simulink model "task1"  (R2022b)
settings: Solver=ode45  StartTime=0.0  StopTime=stoptime  MaxStep=0.01  RelTol=1e-7
values from neighbouring files (symbols this model uses):
  A0 = [1 0 0; 0 1 0; 0 0 1]    [lab6task1m.m]    (also in lab6task2m.m; task1main.m; task2main.m; taskmain.m = vrrotvec2mat(axisangle))
  euler312_0 = [-atan2(A0(2,1),A0(2,2)); asin(A0(2,3)); -atan2(A0(1,3),A0(3,3))]    [lab6task1m.m]    (also in lab6task2m.m; task1main.m; task2main.m; taskmain.m)
  euler313_0 = [-atan2(A0(3,1),A0(3,2)); asin(A0(3,3)); atan2(A0(1,3),A0(2,3))]    [lab6task1m.m]    (also in lab6task2m.m; task1main.m; task2main.m; taskmain.m)
  gamma0 = [0;0;1]    [lab6task1m.m]    (also in lab6task2m.m; task1main.m; task2main.m; taskmain.m = [1;0;0])
  I = diag(I)    [lab6task1m.m]    (also in lab6task2m.m; task1main.m; task2main.m; taskmain.m)
  I_inv = pinv(I)    [lab6task1m.m]    (also in lab6task2m.m; task1main.m; task2main.m; taskmain.m)
  Ir = 0.005    [lab6task1m.m]    (also in lab6task2m.m; task1main.m; task2main.m; taskmain.m)
  k = [0;0;1]    [lab6task1m.m]    (also in lab6task2m.m; task1main.m; task2main.m; taskmain.m)
  M = [0;0;0]    [lab6task1m.m]    (also in lab6task2m.m; task1main.m; task2main.m; taskmain.m)
  Mr = 0    [lab6task1m.m]    (also in lab6task2m.m; task1main.m; task2main.m; taskmain.m)
  n = sqrt(mu_E/(height+R_E)^3)    [lab6task1m.m]    (also in lab6task2m.m; task1main.m; task2main.m)
  q0 = zeros(4,1)    [lab6task1m.m]    (also in lab6task2m.m; task1main.m; task2main.m; taskmain.m)
  w0 = cat(1,w0,wr0)    [lab6task1m.m]    (also in lab6task2m.m; task1main.m; task2main.m; taskmain.m)
  w_LN = [0;0;n]    [lab6task1m.m]    (also in lab6task2m.m; task1main.m; task2main.m)
libraries: matrix_library x3, vrlib x2
settings Model: Creator=a1pab  LastModifiedBy=a1pab

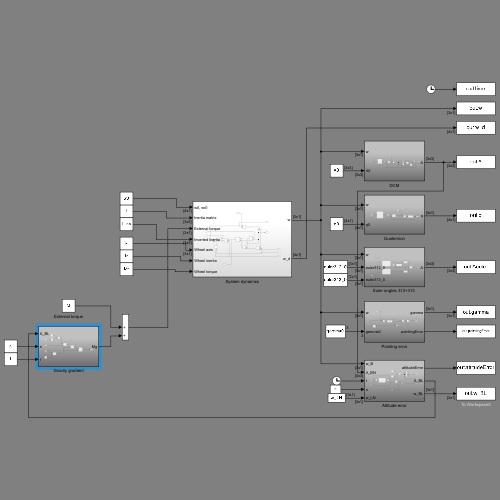
[thumbnail: Simulink's stored preview of the top-level diagram]
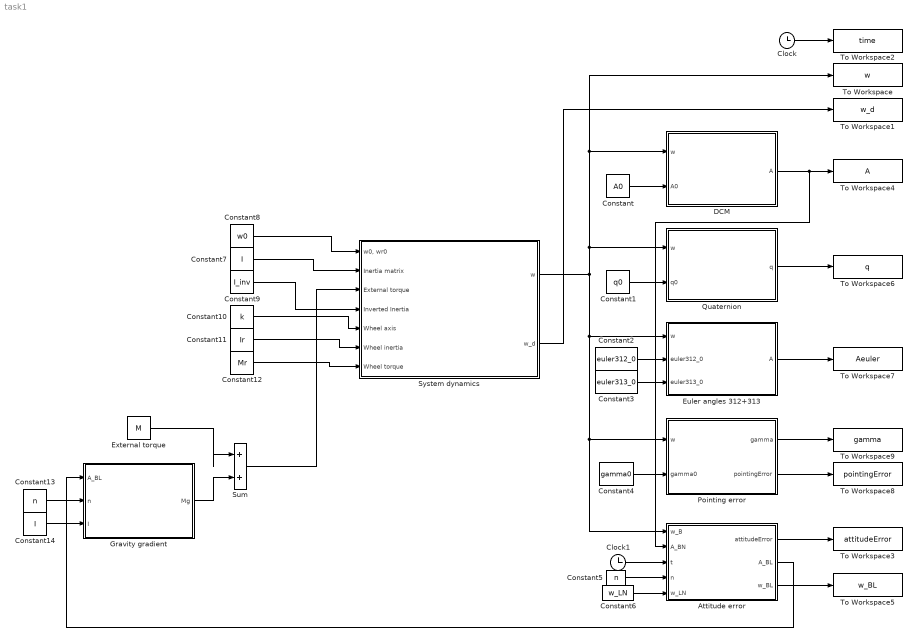
== system task1 ==
  Attitude error : Subsystem
  Clock : Clock
  Clock1 : Clock
  Constant : Constant  Value=A0  VectorParams1D=off
  Constant1 : Constant  Value=q0  VectorParams1D=off
  Constant10 : Constant  Value=k  VectorParams1D=off
  Constant11 : Constant  Value=Ir
  Constant12 : Constant  Value=Mr
  Constant13 : Constant  Value=n  VectorParams1D=off
  Constant14 : Constant  Value=I  VectorParams1D=off
  Constant2 : Constant  Value=euler312_0  VectorParams1D=off
  Constant3 : Constant  Value=euler313_0  VectorParams1D=off
  Constant4 : Constant  Value=gamma0
  Constant5 : Constant  Value=n  VectorParams1D=off
  Constant6 : Constant  Value=w_LN  VectorParams1D=off
  Constant7 : Constant  Value=I  VectorParams1D=off
  Constant8 : Constant  Value=w0  VectorParams1D=off
  Constant9 : Constant  Value=I_inv  VectorParams1D=off
  DCM : Subsystem
  "Euler angles 312+313 " : Subsystem
  External torque : Constant  Value=M
  Gravity gradient : Subsystem
  Pointing error : Subsystem
  Quaternion : Subsystem
  Sum : Sum  Inputs=|++
  System dynamics : Subsystem
  To Workspace : ToWorkspace  VariableName=w  SampleTime=-1
  To Workspace1 : ToWorkspace  VariableName=w_d  SampleTime=-1
  To Workspace2 : ToWorkspace  VariableName=time  SampleTime=-1
  To Workspace3 : ToWorkspace  VariableName=attitudeError  SampleTime=-1
  To Workspace4 : ToWorkspace  VariableName=A  SampleTime=-1
  To Workspace5 : ToWorkspace  VariableName=w_BL  SampleTime=-1
  To Workspace6 : ToWorkspace  VariableName=q  SampleTime=-1
  To Workspace7 : ToWorkspace  VariableName=Aeuler  SampleTime=-1
  To Workspace8 : ToWorkspace  VariableName=pointingError  SampleTime=-1
  To Workspace9 : ToWorkspace  VariableName=gamma  SampleTime=-1
  wires:
  System dynamics/1(w) -> Attitude error/1(w_B), Pointing error/1(w), "Euler angles 312+313 "/1(w), Quaternion/1(w), To Workspace/1, DCM/1(w)
  System dynamics/2(w_d) -> To Workspace1/1
  Clock/1 -> To Workspace2/1
  Constant10/1 -> System dynamics/5(Wheel axis)
  Constant11/1 -> System dynamics/6(Wheel inertia)
  Constant12/1 -> System dynamics/7(Wheel torque)
  Constant8/1 -> System dynamics/1("w0, wr0")
  Constant7/1 -> System dynamics/2(Inertia matrix)
  Constant9/1 -> System dynamics/4(Inverted Inertia)
  Constant/1 -> DCM/2(A0)
  Constant1/1 -> Quaternion/2(q0)
  Quaternion/1(q) -> To Workspace6/1
  Constant2/1 -> "Euler angles 312+313 "/2(euler312_0)
  Constant3/1 -> "Euler angles 312+313 "/3(euler313_0)
  "Euler angles 312+313 "/1(A) -> To Workspace7/1
  Constant4/1 -> Pointing error/2(gamma0)
  Pointing error/2(pointingError) -> To Workspace8/1
  Pointing error/1(gamma) -> To Workspace9/1
  DCM/1(A) -> Attitude error/2(A_BN), To Workspace4/1
  Attitude error/1(attitudeError) -> To Workspace3/1
  Attitude error/3(w_BL) -> To Workspace5/1
  Clock1/1 -> Attitude error/3(t)
  Constant5/1 -> Attitude error/4(n)
  Constant6/1 -> Attitude error/5(w_LN)
  External torque/1 -> Sum/1
  Gravity gradient/1(Mg) -> Sum/2
  Sum/1 -> System dynamics/3(External torque)
  Attitude error/2(A_BL) -> Gravity gradient/1(A_BL)
  Constant13/1 -> Gravity gradient/2(n)
  Constant14/1 -> Gravity gradient/3(I)

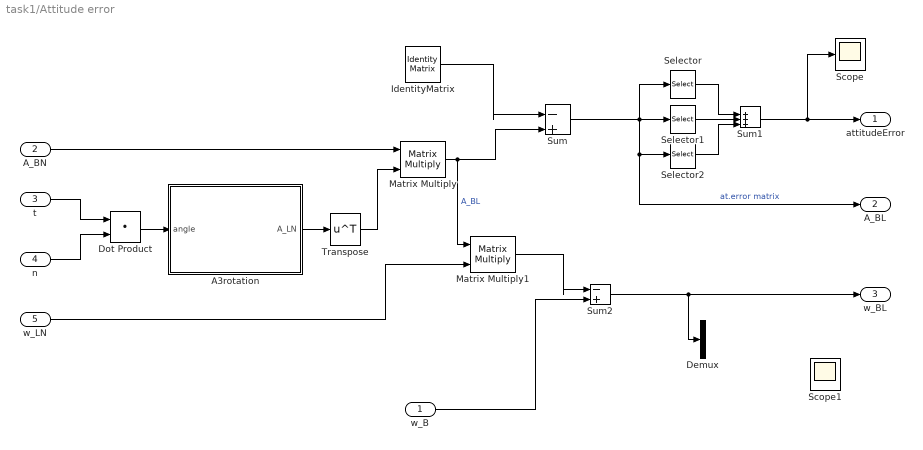
== system task1/Attitude error ==
  w_B : Inport
  A_BN : Inport  Port=2
  t : Inport  Port=3
  n : Inport  Port=4
  w_LN : Inport  Port=5
  A3rotation : Subsystem
  Demux : Demux  Outputs=3
  Dot Product : DotProduct  OutDataTypeStr=Inherit: Inherit via internal rule
  IdentityMatrix : IdentityMatrix  OutputDimensions=3
  Matrix Multiply : Product  Multiplication=Matrix(*)
  Matrix Multiply1 : Product  Multiplication=Matrix(*)
  Scope : Scope
  Scope1 : Scope
  Selector : Selector  NumberOfDimensions=2  InputPortWidth=3  IndexOptions=Index vector (dialog),Index vector (dialog)  Indices=1,1  OutputSizes=1,1
  Selector1 : Selector  NumberOfDimensions=2  InputPortWidth=3  IndexOptions=Index vector (dialog),Index vector (dialog)  Indices=2,2  OutputSizes=1,1
  Selector2 : Selector  NumberOfDimensions=2  InputPortWidth=3  IndexOptions=Index vector (dialog),Index vector (dialog)  Indices=3,3  OutputSizes=1,1
  Sum : Sum  Inputs=|-+
  Sum1 : Sum  Inputs=|+++
  Sum2 : Sum  Inputs=|-+
  Transpose : Math  Operator=transpose
  attitudeError : Outport
  A_BL : Outport  Port=2
  w_BL : Outport  Port=3
  wires:
  t/1 -> Dot Product/1
  n/1 -> Dot Product/2
  Dot Product/1 -> A3rotation/1(angle)
  A3rotation/1(A_LN) -> Transpose/1
  Transpose/1 -> Matrix Multiply/2
  A_BN/1 -> Matrix Multiply/1
  Matrix Multiply/1 -> Matrix Multiply1/1, Sum/2  "A_BL"
  IdentityMatrix/1 -> Sum/1
  Sum/1 -> Selector/1, Selector1/1, A_BL/1, Selector2/1  "at.error matrix"
  Selector/1 -> Sum1/1
  Selector1/1 -> Sum1/2
  Selector2/1 -> Sum1/3
  w_B/1 -> Sum2/2
  Matrix Multiply1/1 -> Sum2/1
  w_LN/1 -> Matrix Multiply1/2
  Sum1/1 -> Scope/1, attitudeError/1
  Sum2/1 -> Demux/1, w_BL/1

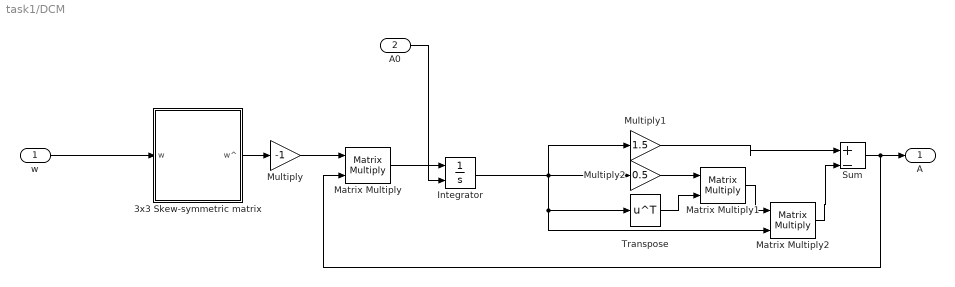
== system task1/DCM ==
  w : Inport
  A0 : Inport  Port=2
  3x3 Skew-symmetric matrix : Subsystem
  Integrator : Integrator  InitialConditionSource=external
  Matrix Multiply : Product  Multiplication=Matrix(*)
  Matrix Multiply1 : Product  Multiplication=Matrix(*)
  Matrix Multiply2 : Product  Multiplication=Matrix(*)
  Multiply : Gain  Gain=-1
  Multiply1 : Gain  Gain=1.5
  Multiply2 : Gain  Gain=0.5
  Sum : Sum  Inputs=|+-
  Transpose : Math  Operator=transpose
  A : Outport
  wires:
  w/1 -> 3x3 Skew-symmetric matrix/1(w)
  3x3 Skew-symmetric matrix/1(w^) -> Multiply/1
  Multiply/1 -> Matrix Multiply/1
  Matrix Multiply/1 -> Integrator/1
  A0/1 -> Integrator/2
  Integrator/1 -> Transpose/1, Matrix Multiply2/2, Multiply2/1, Multiply1/1
  Transpose/1 -> Matrix Multiply1/2
  Sum/1 -> Matrix Multiply/2, A/1
  Matrix Multiply1/1 -> Matrix Multiply2/1
  Matrix Multiply2/1 -> Sum/2
  Multiply1/1 -> Sum/1
  Multiply2/1 -> Matrix Multiply1/1

== system task1/Euler angles 312+313  ==
  w : Inport
  euler312_0 : Inport  Port=2
  euler313_0 : Inport  Port=3
  Abs : Abs  SaturateOnIntegerOverflow=off
  If : If  IfExpression=u1 > 0.1
  If Action Subsystem : Subsystem  TreatAsAtomicUnit=on
  If Action Subsystem1 : Subsystem  TreatAsAtomicUnit=on
  Integrate euler312 : Subsystem
  Integrate euler313 : Subsystem
  Switch : Switch  Criteria=u2 > Threshold  Threshold=0.1  SaturateOnIntegerOverflow=off  InputSameDT=off
  A : Outport
  wires:
  w/1 -> Integrate euler313/1(w), Integrate euler312/1(w)
  euler312_0/1 -> Integrate euler312/2(angles0)
  euler313_0/1 -> Integrate euler313/2(angles0)
  Integrate euler312/2(cos(theta)312) -> Abs/1
  Abs/1 -> Switch/2, If/1
  Integrate euler312/1(euler312) -> If Action Subsystem/1(euler312)
  If/1 -> If Action Subsystem/Action
  Integrate euler313/1(euler313) -> If Action Subsystem1/1(euler313)
  If/2 -> If Action Subsystem1/Action
  If Action Subsystem/1(A) -> Switch/1
  If Action Subsystem1/1(A) -> Switch/3
  Switch/1 -> A/1

== system task1/Gravity gradient ==
  A_BL : Inport
  n : Inport  Port=2
  I : Inport  Port=3
  Constant : Constant  Value=3
  Constant1 : Constant  Value=[1;0;0]  VectorParams1D=off
  Cross Product : matrix_library/Cross Product
  Dot Product : DotProduct  OutDataTypeStr=Inherit: Inherit via internal rule
  Matrix Multiply : Product
  Matrix Multiply1 : Product  Multiplication=Matrix(*)
  Matrix Multiply2 : Product  Multiplication=Matrix(*)
  Square : Math  Operator=square
  Mg : Outport
  wires:
  Constant/1 -> Dot Product/1
  n/1 -> Square/1
  Square/1 -> Dot Product/2
  I/1 -> Matrix Multiply/2
  Dot Product/1 -> Matrix Multiply/1
  Matrix Multiply/1 -> Matrix Multiply1/1
  Matrix Multiply1/1 -> Cross Product/1
  Cross Product/1 -> Mg/1  "3n^2*I*c x c"
  A_BL/1 -> Matrix Multiply2/1
  Constant1/1 -> Matrix Multiply2/2
  Matrix Multiply2/1 -> Cross Product/2, Matrix Multiply1/2  "c"

== system task1/Pointing error ==
  w : Inport
  gamma0 : Inport  Port=2
  Acos : Trigonometry  Operator=acos
  Cross Product : matrix_library/Cross Product
  Dot Product : DotProduct  OutDataTypeStr=Inherit: Inherit via internal rule
  Integrator : Integrator  InitialConditionSource=external
  Normalize Vector : vrlib/Utilities/Normalize Vector  maxzero=0
  gamma : Outport
  pointingError : Outport  Port=2
  wires:
  gamma0/1 -> Dot Product/1, Integrator/2
  w/1 -> Cross Product/2
  Cross Product/1 -> Integrator/1
  Integrator/1 -> Normalize Vector/1
  Normalize Vector/1 -> Dot Product/2, gamma/1, Cross Product/1
  Dot Product/1 -> Acos/1
  Acos/1 -> pointingError/1

== system task1/Quaternion ==
  w : Inport
  q0 : Inport  Port=2
  4x4 Skew-symmetric matrix : Subsystem
  Integrator : Integrator  InitialConditionSource=external
  Matrix Multiply : Product  Multiplication=Matrix(*)
  Multiply : Gain  Gain=0.5
  Normalize Vector : vrlib/Utilities/Normalize Vector  maxzero=0
  q : Outport
  wires:
  w/1 -> 4x4 Skew-symmetric matrix/1(w)
  4x4 Skew-symmetric matrix/1(w^) -> Multiply/1
  Multiply/1 -> Matrix Multiply/1
  Matrix Multiply/1 -> Integrator/1
  q0/1 -> Integrator/2
  Integrator/1 -> Normalize Vector/1
  Normalize Vector/1 -> Matrix Multiply/2, q/1

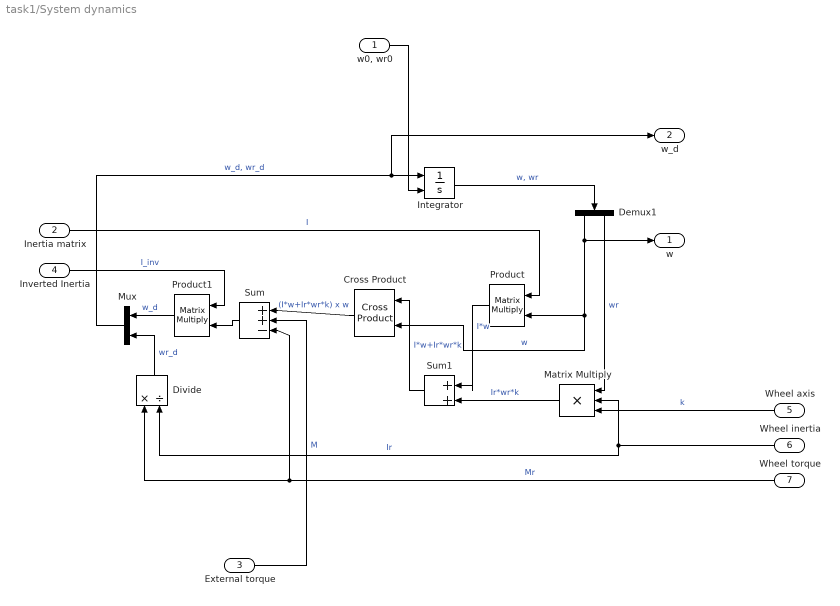
== system task1/System dynamics ==
  "w0, wr0" : Inport
  Inertia matrix : Inport  Port=2
  External torque : Inport  Port=3
  Inverted Inertia : Inport  Port=4
  Wheel axis : Inport  Port=5
  Wheel inertia : Inport  Port=6
  Wheel torque : Inport  Port=7
  Cross Product : matrix_library/Cross Product
  Demux1 : Demux  Outputs=2
  Divide : Product  Inputs=*/
  Integrator : Integrator  InitialConditionSource=external
  Matrix Multiply : Product  Inputs=3
  Mux : Mux  Inputs=2
  Product : Product  Multiplication=Matrix(*)
  Product1 : Product  Multiplication=Matrix(*)
  Sum : Sum  Inputs=|++-
  Sum1 : Sum  Inputs=|++
  w : Outport
  w_d : Outport  Port=2
  wires:
  Mux/1 -> w_d/1, Integrator/1  "w_d, wr_d"
  Integrator/1 -> Demux1/1  "w, wr"
  "w0, wr0"/1 -> Integrator/2
  Product/1 -> Sum1/1  "I*w"
  Cross Product/1 -> Sum/1  "(I*w+Ir*wr*k) x w"
  Inverted Inertia/1 -> Product1/1  "I_inv"
  Inertia matrix/1 -> Product/1  "I"
  Sum/1 -> Product1/2
  External torque/1 -> Sum/2  "M"
  Product1/1 -> Mux/1  "w_d"
  Wheel torque/1 -> Sum/3, Divide/1  "Mr"
  Wheel inertia/1 -> Divide/2, Matrix Multiply/2  "Ir"
  Divide/1 -> Mux/2  "wr_d"
  Demux1/1 -> w/1, Product/2, Cross Product/2  "w"
  Sum1/1 -> Cross Product/1  "I*w+Ir*wr*k"
  Demux1/2 -> Matrix Multiply/1  "wr"
  Matrix Multiply/1 -> Sum1/2  "Ir*wr*k"
  Wheel axis/1 -> Matrix Multiply/3  "k"

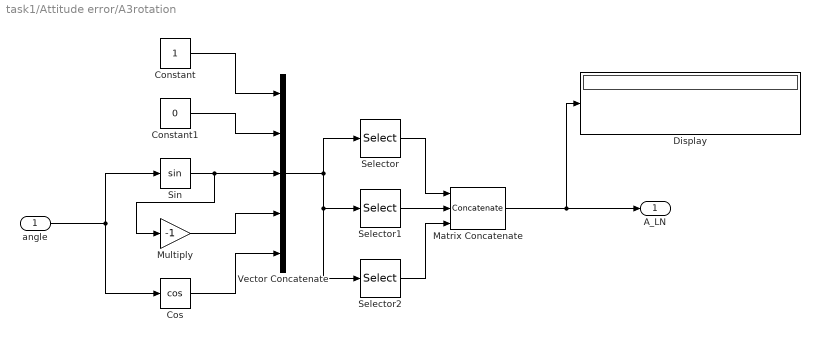
== system task1/Attitude error/A3rotation ==
  angle : Inport
  Constant : Constant
  Constant1 : Constant  Value=0
  Cos : Trigonometry  Operator=cos
  Display : Display
  Matrix Concatenate : Concatenate  NumInputs=3  Mode=Multidimensional array  ConcatenateDimension=2
  Multiply : Gain  Gain=-1
  Selector : Selector  InputPortWidth=5  IndexOptions=Index vector (dialog)  Indices=[5 4 2]  OutputSizes=1
  Selector1 : Selector  InputPortWidth=5  IndexOptions=Index vector (dialog)  Indices=[3 5 2]  OutputSizes=1
  Selector2 : Selector  InputPortWidth=5  IndexOptions=Index vector (dialog)  Indices=[2 2 1]  OutputSizes=1
  Sin : Trigonometry
  Vector Concatenate : Concatenate  NumInputs=5
  A_LN : Outport
  wires:
  angle/1 -> Cos/1, Sin/1
  Sin/1 -> Vector Concatenate/3, Multiply/1
  Constant/1 -> Vector Concatenate/1
  Constant1/1 -> Vector Concatenate/2
  Multiply/1 -> Vector Concatenate/4
  Cos/1 -> Vector Concatenate/5
  Vector Concatenate/1 -> Selector2/1, Selector1/1, Selector/1
  Selector/1 -> Matrix Concatenate/1
  Selector1/1 -> Matrix Concatenate/2
  Selector2/1 -> Matrix Concatenate/3
  Matrix Concatenate/1 -> Display/1, A_LN/1

== system task1/DCM/3x3 Skew-symmetric matrix ==
  w : Inport
  Constant : Constant  Value=0
  Display : Display
  Matrix Concatenate : Concatenate  NumInputs=3  Mode=Multidimensional array  ConcatenateDimension=2
  Multiply : Gain  Gain=-1
  Scope : Scope
  Selector : Selector  InputPortWidth=7  IndexOptions=Index vector (dialog)  Indices=[4 1 5]  OutputSizes=1
  Selector1 : Selector  InputPortWidth=7  IndexOptions=Index vector (dialog)  Indices=[1 7 3]  OutputSizes=1
  Selector2 : Selector  InputPortWidth=7  IndexOptions=Index vector (dialog)  Indices=[6 2 1]  OutputSizes=1
  Transpose : Math  Operator=transpose
  Vector Concatenate : Concatenate  NumInputs=3
  w^ : Outport
  wires:
  Matrix Concatenate/1 -> Transpose/1
  Selector/1 -> Matrix Concatenate/2
  Selector2/1 -> Matrix Concatenate/3
  Selector1/1 -> Matrix Concatenate/1
  Vector Concatenate/1 -> Selector2/1, Selector/1, Selector1/1
  Constant/1 -> Vector Concatenate/1
  w/1 -> Scope/1, Multiply/1, Vector Concatenate/2
  Multiply/1 -> Vector Concatenate/3  "-w"
  Transpose/1 -> Display/1, w^/1

== system task1/Euler angles 312+313 /If Action Subsystem ==
  euler312 : Inport
  Action Port : ActionPort  ActionPortLabel=if(u1 > 0.1)
  A1rotation : Subsystem
  A2rotation : Subsystem
  A3rotation : Subsystem
  Demux : Demux  Outputs=3
  Display : Display
  Matrix Multiply : Product  Inputs=3  Multiplication=Matrix(*)
  A : Outport
  wires:
  euler312/1 -> Demux/1
  Matrix Multiply/1 -> Display/1, A/1
  A2rotation/1(matrix) -> Matrix Multiply/1
  A1rotation/1(matrix) -> Matrix Multiply/2
  A3rotation/1(matrix) -> Matrix Multiply/3
  Demux/1 -> A3rotation/1(angle)
  Demux/2 -> A1rotation/1(angle)
  Demux/3 -> A2rotation/1(angle)

== system task1/Euler angles 312+313 /If Action Subsystem1 ==
  euler313 : Inport
  Action Port : ActionPort  ActionPortLabel=else
  A1rotation : Subsystem
  A3rotation : Subsystem
  A3rotation1 : Subsystem
  Demux : Demux  Outputs=3
  Display : Display
  Matrix Multiply : Product  Inputs=3  Multiplication=Matrix(*)
  A : Outport
  wires:
  euler313/1 -> Demux/1
  A1rotation/1(matrix) -> Matrix Multiply/2
  A3rotation1/1(matrix) -> Matrix Multiply/1
  A3rotation/1(matrix) -> Matrix Multiply/3
  Matrix Multiply/1 -> A/1, Display/1
  Demux/1 -> A3rotation/1(angle)
  Demux/2 -> A1rotation/1(angle)
  Demux/3 -> A3rotation1/1(angle)

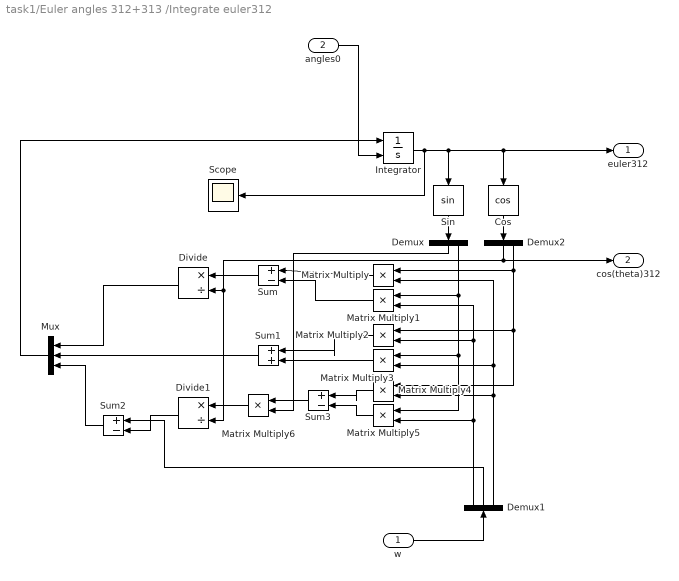
== system task1/Euler angles 312+313 /Integrate euler312 ==
  w : Inport
  angles0 : Inport  Port=2
  Cos : Trigonometry  Operator=cos
  Demux : Demux  Outputs=3
  Demux1 : Demux  Outputs=3
  Demux2 : Demux  Outputs=3
  Divide : Product  Inputs=*/
  Divide1 : Product  Inputs=*/
  Integrator : Integrator  InitialConditionSource=external
  Matrix Multiply{,1..6} (7 alike) : Product
  Mux : Mux  Inputs=3
  Scope : Scope
  Sin : Trigonometry
  Sum : Sum  Inputs=|+-
  Sum1 : Sum  Inputs=|++
  Sum2 : Sum  Inputs=|+-
  Sum3 : Sum  Inputs=|+-
  euler312 : Outport
  cos(theta)312 : Outport  Port=2
  wires:
  w/1 -> Demux1/1
  angles0/1 -> Integrator/2
  Integrator/1 -> Scope/1, Sin/1, Cos/1, euler312/1
  Mux/1 -> Integrator/1
  Sin/1 -> Demux/1
  Cos/1 -> Demux2/1
  Demux1/3 -> Matrix Multiply4/2, Matrix Multiply3/2, Matrix Multiply/2
  Demux2/3 -> Matrix Multiply4/1, Matrix Multiply2/1, Matrix Multiply/1
  Matrix Multiply/1 -> Sum/1
  Demux1/1 -> Matrix Multiply5/2, Matrix Multiply2/2, Matrix Multiply1/2
  Demux/3 -> Matrix Multiply5/1, Matrix Multiply3/1, Matrix Multiply1/1
  Matrix Multiply1/1 -> Sum/2
  Sum/1 -> Divide/1
  Divide/1 -> Mux/1
  Demux2/2 -> cos(theta)312/1, Divide1/2, Divide/2
  Matrix Multiply2/1 -> Sum1/1
  Matrix Multiply3/1 -> Sum1/2
  Sum1/1 -> Mux/2
  Sum2/1 -> Mux/3
  Matrix Multiply4/1 -> Sum3/1
  Matrix Multiply5/1 -> Sum3/2
  Sum3/1 -> Matrix Multiply6/1
  Demux/2 -> Matrix Multiply6/2
  Matrix Multiply6/1 -> Divide1/1
  Divide1/1 -> Sum2/2
  Demux1/2 -> Sum2/1

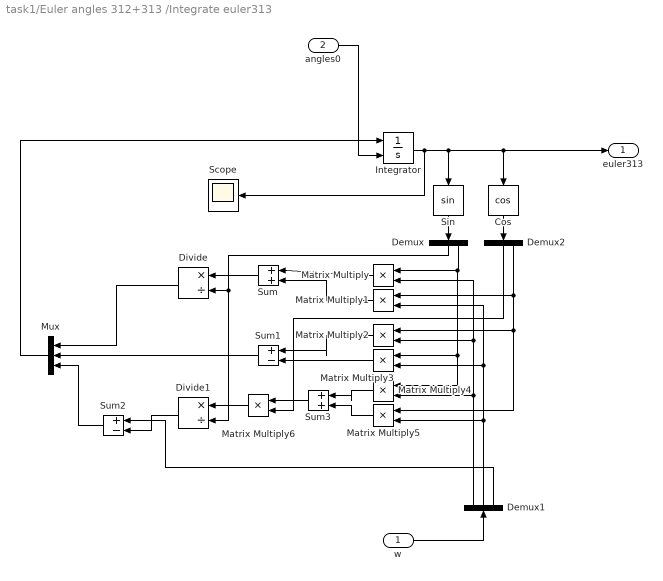
== system task1/Euler angles 312+313 /Integrate euler313 ==
  w : Inport
  angles0 : Inport  Port=2
  Cos : Trigonometry  Operator=cos
  Demux : Demux  Outputs=3
  Demux1 : Demux  Outputs=3
  Demux2 : Demux  Outputs=3
  Divide : Product  Inputs=*/
  Divide1 : Product  Inputs=*/
  Integrator : Integrator  InitialConditionSource=external
  Matrix Multiply{,1..6} (7 alike) : Product
  Mux : Mux  Inputs=3
  Scope : Scope
  Sin : Trigonometry
  Sum : Sum  Inputs=|++
  Sum1 : Sum  Inputs=|+-
  Sum2 : Sum  Inputs=|+-
  Sum3 : Sum  Inputs=|++
  euler313 : Outport
  wires:
  w/1 -> Demux1/1
  Cos/1 -> Demux2/1
  angles0/1 -> Integrator/2
  Sin/1 -> Demux/1
  Integrator/1 -> Scope/1, Sin/1, euler313/1, Cos/1
  Mux/1 -> Integrator/1
  Demux1/1 -> Matrix Multiply4/2, Matrix Multiply2/2, Matrix Multiply/2
  Matrix Multiply/1 -> Sum/1
  Matrix Multiply1/1 -> Sum/2
  Demux1/2 -> Matrix Multiply5/2, Matrix Multiply3/2, Matrix Multiply1/2
  Demux2/3 -> Matrix Multiply5/1, Matrix Multiply2/1, Matrix Multiply1/1
  Sum/1 -> Divide/1
  Demux/2 -> Divide1/2, Divide/2
  Divide/1 -> Mux/1
  Matrix Multiply2/1 -> Sum1/1
  Matrix Multiply3/1 -> Sum1/2
  Sum1/1 -> Mux/2
  Demux/3 -> Matrix Multiply4/1, Matrix Multiply3/1, Matrix Multiply/1
  Matrix Multiply4/1 -> Sum3/1
  Matrix Multiply5/1 -> Sum3/2
  Sum3/1 -> Matrix Multiply6/1
  Demux2/2 -> Matrix Multiply6/2
  Matrix Multiply6/1 -> Divide1/1
  Divide1/1 -> Sum2/2
  Demux1/3 -> Sum2/1
  Sum2/1 -> Mux/3

== system task1/Quaternion/4x4 Skew-symmetric matrix ==
  w : Inport
  Constant : Constant  Value=0
  Display : Display
  Matrix Concatenate : Concatenate  NumInputs=4  Mode=Multidimensional array  ConcatenateDimension=2
  Multiply : Gain  Gain=-1
  Selector : Selector  InputPortWidth=7  IndexOptions=Index vector (dialog)  Indices=[7 1 2 3]  OutputSizes=1
  Selector1 : Selector  InputPortWidth=7  IndexOptions=Index vector (dialog)  Indices=[1 4 6 2]  OutputSizes=1
  Selector2 : Selector  InputPortWidth=7  IndexOptions=Index vector (dialog)  Indices=[3 5 1 4]  OutputSizes=1
  Selector3 : Selector  InputPortWidth=7  IndexOptions=Index vector (dialog)  Indices=[5 6 7 1]  OutputSizes=1
  Transpose : Math  Operator=transpose
  Vector Concatenate : Concatenate  NumInputs=3
  w^ : Outport
  wires:
  Matrix Concatenate/1 -> Transpose/1
  Selector/1 -> Matrix Concatenate/2
  Selector2/1 -> Matrix Concatenate/3
  Selector1/1 -> Matrix Concatenate/1
  Vector Concatenate/1 -> Selector3/1, Selector2/1, Selector/1, Selector1/1
  Constant/1 -> Vector Concatenate/1
  w/1 -> Multiply/1, Vector Concatenate/2
  Multiply/1 -> Vector Concatenate/3  "-w"
  Selector3/1 -> Matrix Concatenate/4
  Transpose/1 -> Display/1, w^/1

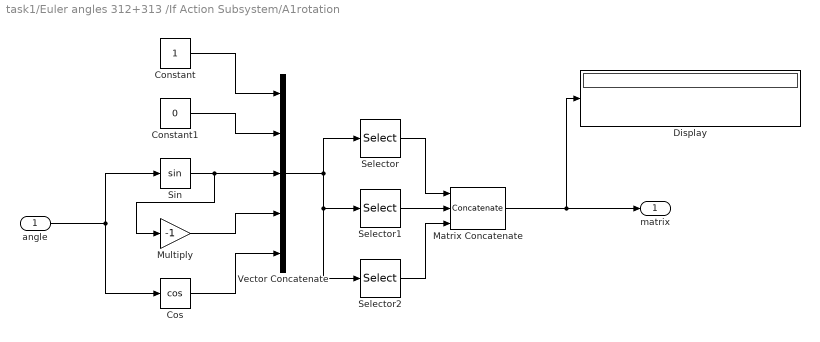
== system task1/Euler angles 312+313 /If Action Subsystem/A1rotation ==
  angle : Inport
  Constant : Constant
  Constant1 : Constant  Value=0
  Cos : Trigonometry  Operator=cos
  Display : Display
  Matrix Concatenate : Concatenate  NumInputs=3  Mode=Multidimensional array  ConcatenateDimension=2
  Multiply : Gain  Gain=-1
  Selector : Selector  InputPortWidth=5  IndexOptions=Index vector (dialog)  Indices=[1 2 2]  OutputSizes=1
  Selector1 : Selector  InputPortWidth=5  IndexOptions=Index vector (dialog)  Indices=[2 5 4]  OutputSizes=1
  Selector2 : Selector  InputPortWidth=5  IndexOptions=Index vector (dialog)  Indices=[2 3 5]  OutputSizes=1
  Sin : Trigonometry
  Vector Concatenate : Concatenate  NumInputs=5
  matrix : Outport
  wires:
  angle/1 -> Cos/1, Sin/1
  Sin/1 -> Vector Concatenate/3, Multiply/1
  Constant/1 -> Vector Concatenate/1
  Constant1/1 -> Vector Concatenate/2
  Multiply/1 -> Vector Concatenate/4
  Cos/1 -> Vector Concatenate/5
  Vector Concatenate/1 -> Selector2/1, Selector1/1, Selector/1
  Selector/1 -> Matrix Concatenate/1
  Selector1/1 -> Matrix Concatenate/2
  Selector2/1 -> Matrix Concatenate/3
  Matrix Concatenate/1 -> Display/1, matrix/1

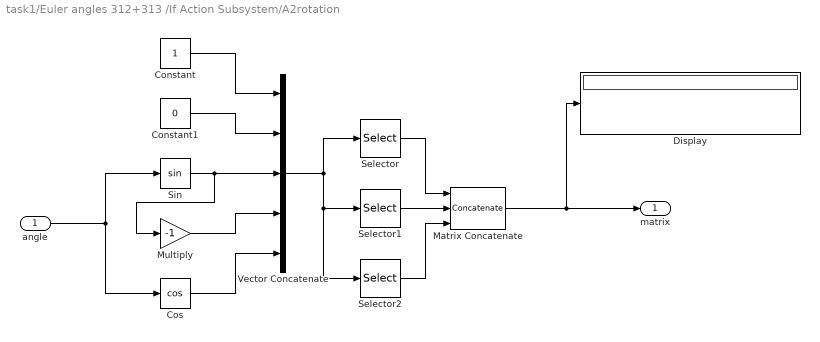
== system task1/Euler angles 312+313 /If Action Subsystem/A2rotation ==
  angle : Inport
  Constant : Constant
  Constant1 : Constant  Value=0
  Cos : Trigonometry  Operator=cos
  Display : Display
  Matrix Concatenate : Concatenate  NumInputs=3  Mode=Multidimensional array  ConcatenateDimension=2
  Multiply : Gain  Gain=-1
  Selector : Selector  InputPortWidth=5  IndexOptions=Index vector (dialog)  Indices=[5 2 3]  OutputSizes=1
  Selector1 : Selector  InputPortWidth=5  IndexOptions=Index vector (dialog)  Indices=[2 1 2]  OutputSizes=1
  Selector2 : Selector  InputPortWidth=5  IndexOptions=Index vector (dialog)  Indices=[4 2 5]  OutputSizes=1
  Sin : Trigonometry
  Vector Concatenate : Concatenate  NumInputs=5
  matrix : Outport
  wires:
  angle/1 -> Cos/1, Sin/1
  Sin/1 -> Vector Concatenate/3, Multiply/1
  Constant/1 -> Vector Concatenate/1
  Constant1/1 -> Vector Concatenate/2
  Multiply/1 -> Vector Concatenate/4
  Cos/1 -> Vector Concatenate/5
  Vector Concatenate/1 -> Selector2/1, Selector1/1, Selector/1
  Selector/1 -> Matrix Concatenate/1
  Selector1/1 -> Matrix Concatenate/2
  Selector2/1 -> Matrix Concatenate/3
  Matrix Concatenate/1 -> Display/1, matrix/1

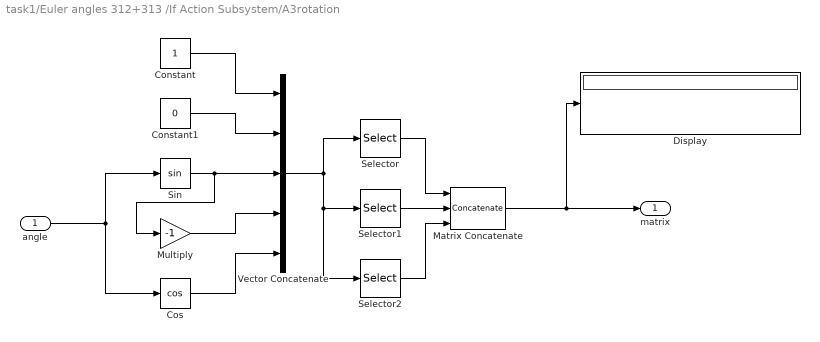
== system task1/Euler angles 312+313 /If Action Subsystem/A3rotation ==
  angle : Inport
  Constant : Constant
  Constant1 : Constant  Value=0
  Cos : Trigonometry  Operator=cos
  Display : Display
  Matrix Concatenate : Concatenate  NumInputs=3  Mode=Multidimensional array  ConcatenateDimension=2
  Multiply : Gain  Gain=-1
  Selector : Selector  InputPortWidth=5  IndexOptions=Index vector (dialog)  Indices=[5 4 2]  OutputSizes=1
  Selector1 : Selector  InputPortWidth=5  IndexOptions=Index vector (dialog)  Indices=[3 5 2]  OutputSizes=1
  Selector2 : Selector  InputPortWidth=5  IndexOptions=Index vector (dialog)  Indices=[2 2 1]  OutputSizes=1
  Sin : Trigonometry
  Vector Concatenate : Concatenate  NumInputs=5
  matrix : Outport
  wires:
  angle/1 -> Cos/1, Sin/1
  Sin/1 -> Vector Concatenate/3, Multiply/1
  Constant/1 -> Vector Concatenate/1
  Constant1/1 -> Vector Concatenate/2
  Multiply/1 -> Vector Concatenate/4
  Cos/1 -> Vector Concatenate/5
  Vector Concatenate/1 -> Selector2/1, Selector1/1, Selector/1
  Selector/1 -> Matrix Concatenate/1
  Selector1/1 -> Matrix Concatenate/2
  Selector2/1 -> Matrix Concatenate/3
  Matrix Concatenate/1 -> Display/1, matrix/1

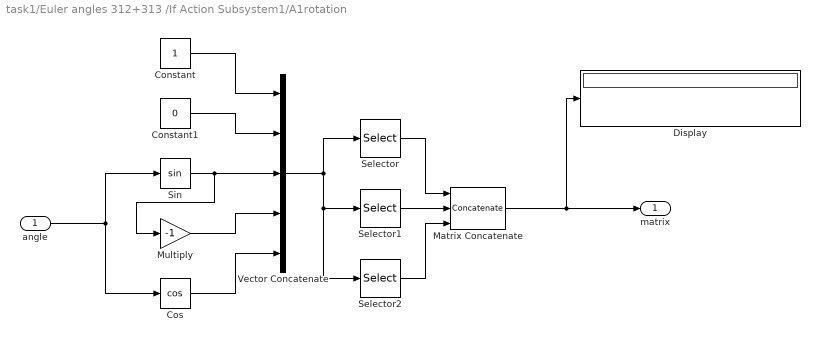
== system task1/Euler angles 312+313 /If Action Subsystem1/A1rotation ==
  angle : Inport
  Constant : Constant
  Constant1 : Constant  Value=0
  Cos : Trigonometry  Operator=cos
  Display : Display
  Matrix Concatenate : Concatenate  NumInputs=3  Mode=Multidimensional array  ConcatenateDimension=2
  Multiply : Gain  Gain=-1
  Selector : Selector  InputPortWidth=5  IndexOptions=Index vector (dialog)  Indices=[1 2 2]  OutputSizes=1
  Selector1 : Selector  InputPortWidth=5  IndexOptions=Index vector (dialog)  Indices=[2 5 4]  OutputSizes=1
  Selector2 : Selector  InputPortWidth=5  IndexOptions=Index vector (dialog)  Indices=[2 3 5]  OutputSizes=1
  Sin : Trigonometry
  Vector Concatenate : Concatenate  NumInputs=5
  matrix : Outport
  wires:
  angle/1 -> Cos/1, Sin/1
  Sin/1 -> Vector Concatenate/3, Multiply/1
  Constant/1 -> Vector Concatenate/1
  Constant1/1 -> Vector Concatenate/2
  Multiply/1 -> Vector Concatenate/4
  Cos/1 -> Vector Concatenate/5
  Vector Concatenate/1 -> Selector2/1, Selector1/1, Selector/1
  Selector/1 -> Matrix Concatenate/1
  Selector1/1 -> Matrix Concatenate/2
  Selector2/1 -> Matrix Concatenate/3
  Matrix Concatenate/1 -> Display/1, matrix/1

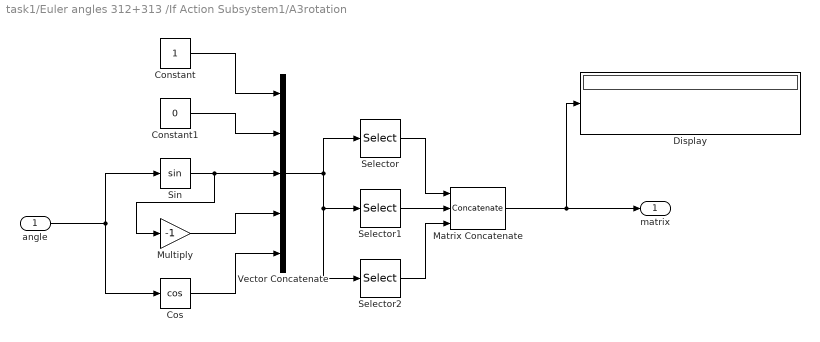
== system task1/Euler angles 312+313 /If Action Subsystem1/A3rotation ==
  angle : Inport
  Constant : Constant
  Constant1 : Constant  Value=0
  Cos : Trigonometry  Operator=cos
  Display : Display
  Matrix Concatenate : Concatenate  NumInputs=3  Mode=Multidimensional array  ConcatenateDimension=2
  Multiply : Gain  Gain=-1
  Selector : Selector  InputPortWidth=5  IndexOptions=Index vector (dialog)  Indices=[5 4 2]  OutputSizes=1
  Selector1 : Selector  InputPortWidth=5  IndexOptions=Index vector (dialog)  Indices=[3 5 2]  OutputSizes=1
  Selector2 : Selector  InputPortWidth=5  IndexOptions=Index vector (dialog)  Indices=[2 2 1]  OutputSizes=1
  Sin : Trigonometry
  Vector Concatenate : Concatenate  NumInputs=5
  matrix : Outport
  wires:
  angle/1 -> Cos/1, Sin/1
  Sin/1 -> Vector Concatenate/3, Multiply/1
  Constant/1 -> Vector Concatenate/1
  Constant1/1 -> Vector Concatenate/2
  Multiply/1 -> Vector Concatenate/4
  Cos/1 -> Vector Concatenate/5
  Vector Concatenate/1 -> Selector2/1, Selector1/1, Selector/1
  Selector/1 -> Matrix Concatenate/1
  Selector1/1 -> Matrix Concatenate/2
  Selector2/1 -> Matrix Concatenate/3
  Matrix Concatenate/1 -> Display/1, matrix/1

== system task1/Euler angles 312+313 /If Action Subsystem1/A3rotation1 ==
  angle : Inport
  Constant : Constant
  Constant1 : Constant  Value=0
  Cos : Trigonometry  Operator=cos
  Display : Display
  Matrix Concatenate : Concatenate  NumInputs=3  Mode=Multidimensional array  ConcatenateDimension=2
  Multiply : Gain  Gain=-1
  Selector : Selector  InputPortWidth=5  IndexOptions=Index vector (dialog)  Indices=[5 4 2]  OutputSizes=1
  Selector1 : Selector  InputPortWidth=5  IndexOptions=Index vector (dialog)  Indices=[3 5 2]  OutputSizes=1
  Selector2 : Selector  InputPortWidth=5  IndexOptions=Index vector (dialog)  Indices=[2 2 1]  OutputSizes=1
  Sin : Trigonometry
  Vector Concatenate : Concatenate  NumInputs=5
  matrix : Outport
  wires:
  angle/1 -> Cos/1, Sin/1
  Sin/1 -> Vector Concatenate/3, Multiply/1
  Constant/1 -> Vector Concatenate/1
  Constant1/1 -> Vector Concatenate/2
  Multiply/1 -> Vector Concatenate/4
  Cos/1 -> Vector Concatenate/5
  Vector Concatenate/1 -> Selector2/1, Selector1/1, Selector/1
  Selector/1 -> Matrix Concatenate/1
  Selector1/1 -> Matrix Concatenate/2
  Selector2/1 -> Matrix Concatenate/3
  Matrix Concatenate/1 -> Display/1, matrix/1
